simulink model "CurrentSystem2019a"  (R2019a)
settings: Solver=ode23tb  StartTime=0  StopTime=24*365*60*60  RelTol=0.1  EnableMultiTasking=on
PreLoadFcn:
  | power_13NodeTestFeeder_init;
undefined symbols (not defined in the file): ABSOLARCap, ABWindCap, BCSOLARCap, BCWindCap, C_601, C_602, C_603, C_604, C_605, C_606, C_607, ft2km, L_601, L_602, L_603, L_604, L_605, L_606, L_607, MBSOLARCap, MBWindCap, NBSOLARCap, NBWindCap, NLSOLARCap, NLWindCap, NSSOLARCap, NSWindCap, NTSOLARCap, NTWindCap, NUSOLARCap, NUWindCap, ONSOLARCap, ONWindCap, PEISOLARCap, PEIWindCap, QCSOLARCap, QCWindCap, R_601, R_602, R_603, R_604, R_605, R_606, R_607, SKSOLARCap, SKWindCap, T_Disconnect, T_Reconnect, Yearsec, YTSOLARCap, YTWindCap
libraries: powerlib_meascontrol x70, powerlib x67, sps_avr x1, spsDieselMotorModel x1
(part 1 of 3)
settings Model: SimulationMode=accelerator  Creator=MathWorks  LastModifiedBy=100618997
settings SolverCC: ZeroCrossControl=DisableAll  ZeroCrossAlgorithm=Adaptive
settings DataIOCC: ExternalInput=getinputstruct(op_IEEE_13_node_5)  InitialState=getstatestruct(op_IEEE_13_node_5)  LimitDataPoints=on  SaveFormat=Array  SaveOutput=off  SignalLogging=off  DSMLogging=off  SaveTime=off  ReturnWorkspaceOutputs=off
settings OptimizationCC: ExpressionDepthLimit=2147483647  EfficientMapNaN2IntZero=off  LifeSpan=inf
settings DebuggingCC: ReadBeforeWriteMsg=DisableAll  WriteAfterWriteMsg=DisableAll  WriteAfterReadMsg=DisableAll  AlgebraicLoopMsg=none  UnderspecifiedInitializationDetection=Classic  MergeDetectMultiDrivingBlocksExec=none  MultiTaskDSMMsg=none  FcnCallInpInsideContextMsg=warning  UnconnectedInputMsg=none  UnconnectedOutputMsg=none  UnconnectedLineMsg=none  AllowSymbolicDim=off  StateNameClashWarn=warning  SFUnexpectedBacktrackingDiag=warning  SFNoUnconditionalDefaultTransitionDiag=warning  SFExecutionAtInitializationDiag=none  ArithmeticOperatorsInVariantConditions=warning
settings HardwareCC: ProdBitPerPointer=32  ProdBitPerSizeT=32  ProdBitPerPtrDiffT=32  ProdLargestAtomicFloat=None  ProdIntDivRoundTo=Undefined  ProdEndianess=Unspecified  ProdWordSize=32  ProdHWDeviceType=32-bit Generic  TargetBitPerPointer=64  TargetBitPerSizeT=64  TargetBitPerPtrDiffT=64  TargetLongLongMode=on  TargetIntDivRoundTo=Zero  TargetEndianess=LittleEndian  TargetWordSize=64  TargetHWDeviceType=MATLAB Host  ProdEqTarget=off
settings ModelReferenceCC: PropagateSignalLabelsOutOfModel=off
settings SFSimCC: SFSimEcho=off  SimUseLocalCustomCode=off
settings CodeAppCC: MaxIdLength=128
settings GRTTargetCC: TargetLangStandard=C89/C90 (ANSI)  GRTInterface=on
settings ConfigComp: CovMetricSettings=dw  CovHtmlReporting=on  CovSaveCumulativeToWorkspaceVar=on  CovSaveSingleToWorkspaceVar=on  CovExternalEMLEnable=off  CovSFcnEnable=off
settings SimscapeCC: SimscapeNormalizeSystem=off

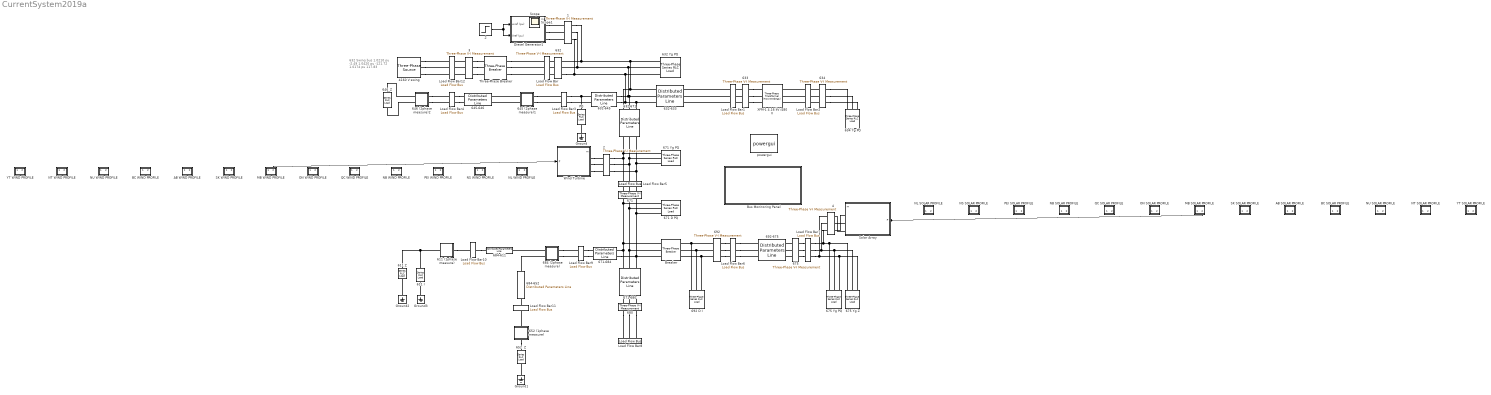
== system CurrentSystem2019a ==
  note: 632 Swing bus
      | 1.0210 pu -2.49
      | 1.0420 pu -121.72
      | 1.0174 pu 117.83
  " 634 Yg PQ " : powerlib/Elements/Three-Phase Series RLC Load  LConnTagsString=A|B|C  Configuration=Y (grounded)  NominalVoltage=120e3  Vabc=[ 0.991722 1.02022 0.993738]*277.128  Vabcp=[1e3 1e3 1e3]  NominalFrequency=60  UnbalancedPower=on  ActivePower=1e+006  InductivePower=0  CapacitivePower=0  Pabc=[160 120 120]*1e3  QLabc=[110 90 90]*1e3  QCabc=[0 0 0]  Pabcp=[10e3 9e3 11e3]  QLabcp=[100 90 110]  QCabcp=[100 90 110]  Measurements=None  LoadType=constant PQ
      settings: SourceProductName=Simscape Electrical
      settings: AttributesFormatString=|
      | P= %<Pabc> W
      | Ql=%<QLabc> var
      | Qc=%<QCabc> var
  .2 : Step  Time=T_Reconnect  Before=1  After=0  SampleTime=0
  1 : powerlib/Measurements/Three-Phase V-I Measurement  VoltageMeasurement=phase-to-ground  SetLabelV=on  LabelV=Vdiesel  Vpu=off  VpuLL=off  CurrentMeasurement=yes  SetLabelI=on  LabelI=Idiesel  Ipu=off  Pbase=100e6  Vbase=4160  OutputType=Complex  PhasorSimulation=on  PSBequivalent=0
      settings: SourceProductName=Simscape Electrical
  2 : powerlib/Measurements/Three-Phase V-I Measurement  VoltageMeasurement=phase-to-ground  SetLabelV=on  LabelV=Vwind  Vpu=off  VpuLL=off  CurrentMeasurement=yes  SetLabelI=on  LabelI=Iwind  Ipu=off  Pbase=100e6  Vbase=4160  OutputType=Complex  PhasorSimulation=on  PSBequivalent=0
      settings: SourceProductName=Simscape Electrical
  3 : powerlib/Measurements/Three-Phase V-I Measurement  VoltageMeasurement=phase-to-ground  SetLabelV=on  LabelV=Vmaingrid  Vpu=off  VpuLL=off  CurrentMeasurement=yes  SetLabelI=on  LabelI=Imaingrid  Ipu=off  Pbase=100e6  Vbase=4160  OutputType=Complex  PhasorSimulation=on  PSBequivalent=0
      settings: SourceProductName=Simscape Electrical
  4 : powerlib/Measurements/Three-Phase V-I Measurement  VoltageMeasurement=phase-to-ground  SetLabelV=on  LabelV=Vsolar  Vpu=off  VpuLL=off  CurrentMeasurement=yes  SetLabelI=on  LabelI=Isolar  Ipu=off  Pbase=100e6  Vbase=4160  OutputType=Complex  PhasorSimulation=on  PSBequivalent=0
      settings: SourceProductName=Simscape Electrical
  4160 V swing : powerlib/Electrical Sources/Three-Phase Source  InternalConnection=Yg  VoltagePhases=on  Voltage=120e3  PhaseAngle=0  Voltage_phases=[ 1.021 1.042 1.0174]*2401.78  PhaseAngles_phases=[ -2.49 -121.72 117.83]  Frequency=60  NonIdealSource=off  SpecifyImpedance=on  Resistance=0.8929  Inductance=16.58e-3  ShortCircuitLevel=100e6  BaseVoltage=120e3  XRratio=10  BusType=swing  Pref=0  Qref=0  Prefabc=[1 1 1]*1e6  Qrefabc=[0 0 0]  Qmin="[-inf  -inf -inf]"  Qmax="[inf  inf inf]"
      settings: SourceProductName=Simscape Electrical
  611 (1phase measure) : Subsystem
  611 I : powerlib/Elements/Series RLC Load  LConnTagsString=a  RConnTagsString=__new0  NominalVoltage=0.985825*2401.78  NominalFrequency=60  ActivePower=170e3  InductivePower=80e3  CapacitivePower=0  Setx0=off  InitialVoltage=0  SetiL0=off  InitialCurrent=0  Measurements=Branch voltage and current  LoadType=constant I
      settings: SourceProductName=Simscape Electrical
      settings: AttributesFormatString=|
      | P=%<ActivePower> W
      | Ql=%<InductivePower> var
      | Qc=%<CapacitivePower> var
  611 Z : powerlib/Elements/Series RLC Load  LConnTagsString=a  RConnTagsString=__new0  NominalVoltage=4160/sqrt(3)  NominalFrequency=60  ActivePower=0  InductivePower=0  CapacitivePower=100e3  Setx0=off  InitialVoltage=0  SetiL0=off  InitialCurrent=0  Measurements=None  LoadType=constant Z
      settings: SourceProductName=Simscape Electrical
      settings: AttributesFormatString=|
      | P=%<ActivePower> W
      | Ql=%<InductivePower> var
      | Qc=%<CapacitivePower> var
  632 : powerlib/Measurements/Three-Phase V-I Measurement  VoltageMeasurement=phase-to-ground  SetLabelV=on  LabelV=Vabc_632  Vpu=off  VpuLL=off  CurrentMeasurement=yes  SetLabelI=on  LabelI=Iabc_632  Ipu=off  Pbase=100e6  Vbase=4160  OutputType=Complex  PhasorSimulation=on  PSBequivalent=0
      settings: SourceProductName=Simscape Electrical
  632 Yg PQ : powerlib/Elements/Three-Phase Series RLC Load  LConnTagsString=A|B|C  Configuration=Y (grounded)  NominalVoltage=120e3  Vabc=[ 1.01897 1.04044 1.01532]*2401.78  Vabcp=[1e3 1e3 1e3]  NominalFrequency=60  UnbalancedPower=on  ActivePower=1e+006  InductivePower=0  CapacitivePower=0  Pabc="[17 66  117]*1e3/2"  QLabc="[10 38  68]*1e3/2"  QCabc=[0 0 0]  Pabcp=[10e3 9e3 11e3]  QLabcp=[100 90 110]  QCabcp=[100 90 110]  Measurements=None  LoadType=constant PQ
      settings: SourceProductName=Simscape Electrical
      settings: AttributesFormatString=|
      | P= %<Pabc> W
      | Ql=%<QLabc> var
      | Qc=%<QCabc> var
  632-633 : powerlib/Elements/Distributed Parameters Line  Phases=3  Frequency=60  Resistance=R_602  Inductance=L_602  Capacitance=C_602  Length=500*ft2km  x1=[501.298249556744 4241.38280163391 4282.12708189344;376.991118430775 376.991118430775 376.991118430775;-2.2614148733286 -0.34157510745785 -1.9168137180942]  x2=[504.588684561712 4230.72062513662 4271.71287268223;376.991118430775 376.991118430775 376.991118430775;-2.26353543885085 -0.342275768758346 -1.91742725559162]  x3=[16.7674456646186 117.682569324759 103.368907043517;376.991118430775 376.991118430775 376.991118430775;2.65069587435361 2.14578500124131 0.446625957105985]  x4=[16.5551069121651 140.665410457147 120.655553593327;376.991118430775 376.991118430775 376.991118430775;-0.568878729363739 -0.875843142008242 -2.56215385674791]  x5=6.41053351781503e-07  V1=ones(3,3)  V2=ones(3,3)  I1=ones(3,3)  I2=ones(3,3)  nHarmo=1  Measurements=None
      settings: SourceProductName=Simscape Electrical
  632-645 : powerlib/Elements/Distributed Parameters Line  Phases=2  Frequency=60  Resistance=R_603(2:3,2:3)  Inductance=L_603(2:3,2:3)  Capacitance=C_603(2:3,2:3)  Length=500*ft2km  x1=[4264.40256081592 2449.37120000517;376.991118430775 376.991118430775;-1.61351597014441 3.12257330541687]  x2=[4292.15394533527 2455.18167402023;376.991118430775 376.991118430775;-1.614116105248 3.12994263723761]  x3=[213.394300129666 87.8697003438014;376.991118430775 376.991118430775;-2.34443706998439 -2.78105546765574]  x4=[197.96033050634 81.3060039726639;376.991118430775 376.991118430775;0.724911523434161 0.392615068886907]  x5=6.57914367465262e-07  V1=ones(3,3)  V2=ones(3,3)  I1=ones(3,3)  I2=ones(3,3)  nHarmo=1  Measurements=None
      settings: SourceProductName=Simscape Electrical
  632-671 : powerlib/Elements/Distributed Parameters Line  Phases=3  Frequency=60  Resistance=R_601  Inductance=L_601  Capacitance=C_601  Length=2000*ft2km  x1=[411.258072802617 4262.34154212984 4279.413254268;376.991118430775 376.991118430775 376.991118430775;2.58888404049218 0.275850406288993 1.83441514058537]  x2=[346.273446515285 4158.03643956185 4231.93277610758;376.991118430775 376.991118430775 376.991118430775;2.89883497125866 0.262414212273929 1.80030975234441]  x3=[177.438259148728 550.32580669605 566.66947309912;376.991118430775 376.991118430775 376.991118430775;-2.70857378445777 2.65722725515321 -1.37114447017259]  x4=[176.777093380408 575.063462206073 592.863838960838;376.991118430775 376.991118430775 376.991118430775;0.437240559698923 -0.444758677085734 1.77250930915245]  x5=2.51909782126786e-06  V1=ones(3,3)  V2=ones(3,3)  I1=ones(3,3)  I2=ones(3,3)  nHarmo=1  Measurements=None
      settings: SourceProductName=Simscape Electrical
  633 : powerlib/Measurements/Three-Phase V-I Measurement  VoltageMeasurement=phase-to-ground  SetLabelV=on  LabelV=Vabc_633  Vpu=off  VpuLL=off  CurrentMeasurement=yes  SetLabelI=on  LabelI=Iabc_633  Ipu=off  Pbase=100e6  Vbase=4160  OutputType=Complex  PhasorSimulation=on  PSBequivalent=0
      settings: SourceProductName=Simscape Electrical
  634 : powerlib/Measurements/Three-Phase V-I Measurement  VoltageMeasurement=phase-to-ground  SetLabelV=on  LabelV=Vabc_634  Vpu=off  VpuLL=off  CurrentMeasurement=yes  SetLabelI=on  LabelI=Iabc_634  Ipu=off  Pbase=100e6  Vbase=4160  OutputType=Complex  PhasorSimulation=on  PSBequivalent=0
      settings: SourceProductName=Simscape Electrical
  645 (2phase measure)1 : Subsystem
  645-646 : powerlib/Elements/Distributed Parameters Line  Phases=2  Frequency=60  Resistance=R_603(2:3,2:3)  Inductance=L_603(2:3,2:3)  Capacitance=C_603(2:3,2:3)  Length=300*ft2km  x1=[4253.51615943753 2449.23478756666;376.991118430775 376.991118430775;1.53247826718143 3.11934493784883]  x2=[4264.00783705366 2449.21160966797;376.991118430775 376.991118430775;1.53284927772704 3.11937264911809]  x3=[139.76322829713 3.84735914896354;376.991118430775 376.991118430775;1.04719191601338 -3.04482503601123]  x4=[121.315610473818 3.30490803236315;376.991118430775 376.991118430775;-2.17648289094728 2.98054667861466]  x5=3.94748620479157e-07  V1=ones(3,3)  V2=ones(3,3)  I1=ones(3,3)  I2=ones(3,3)  nHarmo=1  Measurements=None
      settings: SourceProductName=Simscape Electrical
  646 (2phase measure)2 : Subsystem
  646_Z : powerlib/Elements/Series RLC Load  LConnTagsString=a  RConnTagsString=__new0  NominalVoltage=4160  NominalFrequency=60  ActivePower=230e3  InductivePower=132e3  CapacitivePower=0  Setx0=off  InitialVoltage=0  SetiL0=off  InitialCurrent=0  Measurements=None  LoadType=constant Z
      settings: SourceProductName=Simscape Electrical
      settings: AttributesFormatString=|
      | P=%<ActivePower> W
      | Ql=%<InductivePower> var
      | Qc=%<CapacitivePower> var
  "652  Z " : powerlib/Elements/Series RLC Load  LConnTagsString=a  RConnTagsString=__new0  NominalVoltage=4160/sqrt(3)  NominalFrequency=60  ActivePower=128e3  InductivePower=86e3  CapacitivePower=0  Setx0=off  InitialVoltage=0  SetiL0=off  InitialCurrent=0  Measurements=None  LoadType=constant Z
      settings: SourceProductName=Simscape Electrical
      settings: AttributesFormatString=|
      | P=%<ActivePower> W
      | Ql=%<InductivePower> var
      | Qc=%<CapacitivePower> var
  652 (1phase measure) : Subsystem
  671 : powerlib/Measurements/Three-Phase V-I Measurement  VoltageMeasurement=phase-to-ground  SetLabelV=on  LabelV=Vabc_671  Vpu=off  VpuLL=off  CurrentMeasurement=yes  SetLabelI=on  LabelI=Iabc_671  Ipu=off  Pbase=100e6  Vbase=4160  OutputType=Complex  PhasorSimulation=on  PSBequivalent=0
      settings: SourceProductName=Simscape Electrical
  671 D PQ : powerlib/Elements/Three-Phase Series RLC Load  LConnTagsString=A|B|C  Configuration=Delta  NominalVoltage=120e3  Vabc="[1  1  1]*120e3/sqrt(3)"  Vabcp=[ 1.73966 1.76988 1.71151]*2401.78  NominalFrequency=60  UnbalancedPower=on  ActivePower=1e+006  InductivePower=0  CapacitivePower=0  Pabc="[17 66  117]*1e3/2"  QLabc="[10 38  68]*1e3/2"  QCabc=[0 0 0]  Pabcp=[385 385 385 ]*1e3  QLabcp=[220 220 220]*1e3  QCabcp="[0  0  0]"  Measurements=Branch voltages and currents  LoadType=constant PQ
      settings: SourceProductName=Simscape Electrical
      settings: AttributesFormatString=|
      | P= %<Pabcp> W
      | Ql=%<QLabcp> var
      | Qc=%<QCabcp> var
  671 Yg PQ : powerlib/Elements/Three-Phase Series RLC Load  LConnTagsString=A|B|C  Configuration=Y (grounded)  NominalVoltage=120e3  Vabc=[ 0.987901 1.05099 0.975851]*2401.78  Vabcp=[1e3 1e3 1e3]  NominalFrequency=60  UnbalancedPower=on  ActivePower=1e+006  InductivePower=0  CapacitivePower=0  Pabc="[17 66  117]*1e3/2"  QLabc="[10 38  68]*1e3/2"  QCabc=[0 0 0]  Pabcp=[10e3 9e3 11e3]  QLabcp=[100 90 110]  QCabcp=[100 90 110]  Measurements=None  LoadType=constant PQ
      settings: SourceProductName=Simscape Electrical
      settings: AttributesFormatString=|
      | P= %<Pabc> W
      | Ql=%<QLabc> var
      | Qc=%<QCabc> var
  671-680 : powerlib/Elements/Distributed Parameters Line  Phases=3  Frequency=60  Resistance=R_601  Inductance=L_601  Capacitance=C_601  Length=1000*ft2km  x1=[346.273446515285 4158.03643956185 4231.93277610758;376.991118430775 376.991118430775 376.991118430775;2.8993098100112 0.262807128835779 1.80070073244037]  x2=[346.273485552757 4158.03676052785 4231.93309956574;376.991118430775 376.991118430775 376.991118430775;2.89930977124762 0.262807101445064 1.80070071123254]  x3=[0.46178374393002 16.4417222910227 13.0406156867181;376.991118430775 376.991118430775 376.991118430775;2.89883495201253 0.262414198558244 1.80030974173376]  x4=[0.461783743355683 16.4417222911636 13.0406156869002;376.991118430775 376.991118430775 376.991118430775;2.89930977111503 0.262807101464808 1.80070071123926]  x5=1.25954891063393e-06  V1=ones(3,3)  V2=ones(3,3)  I1=ones(3,3)  I2=ones(3,3)  nHarmo=1  Measurements=None
      settings: SourceProductName=Simscape Electrical
  671-684 : powerlib/Elements/Distributed Parameters Line  Phases=2  Frequency=60  Resistance=R_604([1 3],[1 3])  Inductance=L_604([1 3],[1 3])  Capacitance=C_604([1 3],[1 3])  Length=300*ft2km  x1=[2317.38621246171 4117.96109624564;376.991118430775 376.991118430775;0.961696703414869 2.54346818296187]  x2=[2319.24198937793 4127.84304358144;376.991118430775 376.991118430775;0.96282674091554 2.54452459092107]  x3=[27.1884655613009 142.758498027598;376.991118430775 376.991118430775;1.03773453761655 2.30448005568221]  x4=[20.4997438318642 122.806338198603;376.991118430775 376.991118430775;-2.07913574984399 -0.876981828337958]  x5=3.94748620479157e-07  V1=ones(3,3)  V2=ones(3,3)  I1=ones(3,3)  I2=ones(3,3)  nHarmo=1  Measurements=None
      settings: SourceProductName=Simscape Electrical
  "675 " : powerlib/Measurements/Three-Phase V-I Measurement  VoltageMeasurement=phase-to-ground  SetLabelV=on  LabelV=Vabc_675  Vpu=off  VpuLL=off  CurrentMeasurement=yes  SetLabelI=on  LabelI=Iabc_675  Ipu=off  Pbase=100e6  Vbase=4160  OutputType=Complex  PhasorSimulation=on  PSBequivalent=0
      settings: SourceProductName=Simscape Electrical
  675 Yg PQ : powerlib/Elements/Three-Phase Series RLC Load  LConnTagsString=A|B|C  Configuration=Y (grounded)  NominalVoltage=120e3  Vabc=[ 0.98146 1.05342 0.973762]*2401.78  Vabcp=[1e3 1e3 1e3]  NominalFrequency=60  UnbalancedPower=on  ActivePower=1e+006  InductivePower=0  CapacitivePower=0  Pabc="[485  68  290]*1e3"  QLabc="[190  60  212]*1e3"  QCabc=[0 0 0]  Pabcp=[10e3 9e3 11e3]  QLabcp=[100 90 110]  QCabcp=[100 90 110]  Measurements=Branch voltages and currents  LoadType=constant PQ
      settings: SourceProductName=Simscape Electrical
      settings: AttributesFormatString=|
      | P= %<Pabc> W
      | Ql=%<QLabc> var
      | Qc=%<QCabc> var
  675 Yg Z : powerlib/Elements/Three-Phase Series RLC Load  LConnTagsString=A|B|C  Configuration=Y (grounded)  NominalVoltage=120e3  Vabc="[1  1  1]*4160/sqrt(3)"  Vabcp=[1e3 1e3 1e3]  NominalFrequency=60  UnbalancedPower=on  ActivePower=1e+006  InductivePower=0  CapacitivePower=0  Pabc=[0 0 0]  QLabc=[0 0 0]  QCabc=[200 200 200]*1e3  Pabcp=[10e3 9e3 11e3]  QLabcp=[100 90 110]  QCabcp=[100 90 110]  Measurements=None  LoadType=constant Z
      settings: SourceProductName=Simscape Electrical
      settings: AttributesFormatString=|
      | P= %<Pabc> W
      | Ql=%<QLabc> var
      | Qc=%<QCabc> var
  680 : powerlib/Measurements/Three-Phase V-I Measurement  VoltageMeasurement=phase-to-ground  SetLabelV=on  LabelV=Vabc_680  Vpu=off  VpuLL=off  CurrentMeasurement=yes  SetLabelI=on  LabelI=Iabc_680  Ipu=off  Pbase=100e6  Vbase=4160  OutputType=Complex  PhasorSimulation=on  PSBequivalent=0
      settings: SourceProductName=Simscape Electrical
  684 (2phase measure) : Subsystem
  684-611 : powerlib/Elements/Distributed Parameters Line  Phases=1  Frequency=60  Resistance=R_605(3,3)  Inductance=L_605(3,3)  Capacitance=C_605(3,3)  Length=300*ft2km  x1=[3314.5063708128;376.991118430775;2.02689942323022]  x2=[3321.32988758383;376.991118430775;2.02944736803624]  x3=[107.053862067257;376.991118430775;2.12194507149989]  x4=[94.9628871920728;376.991118430775;-1.00765726793177]  x5=3.71926621942778e-07  V1=ones(3,3)  V2=ones(3,3)  I1=ones(3,3)  I2=ones(3,3)  nHarmo=1  Measurements=None
      settings: SourceProductName=Simscape Electrical
  684-652 : powerlib/Elements/Distributed Parameters Line  Phases=1  Frequency=60  Resistance=R_607(1,1)  Inductance=L_607(1,1)  Capacitance=C_607(1,1)  Length=800*ft2km  x1=[3364.00980712148;376.991118430775;-0.0876071344539785]  x2=[3345.0390998936;376.991118430775;-0.0863060663875372]  x3=[57.9909734563849;376.991118430775;2.02581298772652]  x4=[128.189096775588;376.991118430775;-0.48531897158013]  x5=2.71396421650751e-06  V1=ones(3,3)  V2=ones(3,3)  I1=ones(3,3)  I2=ones(3,3)  nHarmo=1  Measurements=None
      settings: SourceProductName=Simscape Electrical
  692 : powerlib/Measurements/Three-Phase V-I Measurement  VoltageMeasurement=phase-to-ground  SetLabelV=on  LabelV=Vabc_692  Vpu=off  VpuLL=off  CurrentMeasurement=yes  SetLabelI=on  LabelI=Iabc_692  Ipu=off  Pbase=100e6  Vbase=4160  OutputType=Complex  PhasorSimulation=on  PSBequivalent=0
      settings: SourceProductName=Simscape Electrical
  692 D I : powerlib/Elements/Three-Phase Series RLC Load  LConnTagsString=A|B|C  Configuration=Delta  NominalVoltage=120e3  Vabc="[1  1  1]*120e3/sqrt(3)"  Vabcp=[ 1.73585 1.75086 1.72174]*2401.78  NominalFrequency=60  UnbalancedPower=on  ActivePower=1e+006  InductivePower=0  CapacitivePower=0  Pabc="[17 66  117]*1e3/2"  QLabc="[10 38  68]*1e3/2"  QCabc=[0 0 0]  Pabcp=[1e-6 1e-6 170 ]*1e3  QLabcp=[0 0 151]*1e3  QCabcp="[0  0  0]"  Measurements=Branch voltages and currents  LoadType=constant I
      settings: SourceProductName=Simscape Electrical
      settings: AttributesFormatString=|
      | P= %<Pabcp> W
      | Ql=%<QLabcp> var
      | Qc=%<QCabcp> var
  692-675 : powerlib/Elements/Distributed Parameters Line  Phases=3  Frequency=60  Resistance=R_606  Inductance=L_606  Capacitance=C_606  Length=500*ft2km  x1=[241.289496642843 4129.29083181281 4257.51535779195;376.991118430775 376.991118430775 376.991118430775;-1.71976827629363 2.54633306210785 -2.14602940424835]  x2=[256.665851258922 4119.5124518439 4255.36005403233;376.991118430775 376.991118430775 376.991118430775;-1.79076499561998 2.54378648977405 -2.14685741555792]  x3=[166.881820949653 164.603040297361 23.9250117588126;376.991118430775 376.991118430775 376.991118430775;-2.92243066280774 -0.42985333149663 2.52484844339319]  x4=[164.240261344418 287.086932785949 139.040045332788;376.991118430775 376.991118430775 376.991118430775;0.179837319068752 2.64019694933151 -1.97394240629806]  x5=1.72234634931087e-06  V1=ones(3,3)  V2=ones(3,3)  I1=ones(3,3)  I2=ones(3,3)  nHarmo=1  Measurements=None
      settings: SourceProductName=Simscape Electrical
  AB SOLAR PROFILE : Subsystem
  AB WIND PROFILE : Subsystem
  BC SOLAR PROFILE : Subsystem
  BC WIND PROFILE : Subsystem
  Breaker : powerlib/Elements/Three-Phase Breaker  InitialState=closed  SwitchA=off  SwitchB=off  SwitchC=off  SwitchTimes=[0.5 ]  External=off  BreakerResistance=0.0001  SnubberResistance=inf  SnubberCapacitance=0  Measurements=None
      settings: SourceProductName=Simscape Electrical
  Bus Monitoring Panel : Subsystem
  Diesel Generator1 : Subsystem  mask(Diesel Generator (Simple)){Pn=3e6, Vn=4160, Fn=60, genType=PQ, PQ0=[0 0]}
      mask prompts: Pn "Generator Rated Power [W]"; Vn "Rated Voltage [V]"; Fn "Rated Frequency [Hz]"; genType "Load Flow Type"; PQ0 "Initial Power, [P0 Q0] [pu]"
      mask help:
      | The Diesel Generator block contains a synchronous generator, diesel governor and excitation system to represent the dynamics of a Genset. To inspect the model, look under the block mask (Ctrl + u).
      |
      | The inputs to the basic Diesel generator block are the desired speed reference (in pu) and the desired voltage reference (in pu). The output measurements are contained in a Simulink bus, which can be selected by using the Bus Selector block.
      |
      | Note: The initial generator power must be specified for use for Load Flow analysis.
      mask init:
      | % Extract Initial Active/Reactive Power
      | P0 = PQ0(1);
      | Q0 = PQ0(2);
      | 
      | % Select Load Flow Type
      | genBlock = [gcb '/Synchronous Machine'];
      | currentVals = get_param(genBlock,'MaskValues');
      | currentVals{31} = genType;
      | set_param(genBlock,'MaskValues',currentVals);
      | 
      | % Disable Option if Swing Generator Selected
      | currentEnables = get_param(gcb,'MaskEnables');
      | if strcmp(genType,'swing')
      |     currentEnables{5} = 'off';
      | else
      |     currentEnables{5} = 'on';
      | end
      | set_param(gcb,'MaskEnables',currentEnables);
      settings: AttributesFormatString=Rated Power: %<Pn> W
      mask TypeOptions genType: swing | PQ | PV
      mask Display: %image(imread('diesel.jpg'))
  Ground{,1..3} (4 alike) : powerlib/Elements/Ground  LConnTagsString=a
      settings: SourceProductName=Simscape Electrical
  Load Flow Bar : powerlib/Measurements/Load Flow Bus  LConnTagsString=a|b|c  RConnTagsString=a|b|c  Phases=ABC  Connectors=on both sides  ID=632  Vbase=4160/sqrt(3)  Vref="[ 1.0210  1.0420  1.0174]"  Vangle="[ -2.49  -121.72  117.83]"  VLF=1.019  VLFb=1.04  VLFc=1.015  angleLF=-2.435  angleLFb=-121.7  angleLFc=117.9
      settings: AttributesFormatString=%<ID>  SourceProductName=Simscape Electrical
  Load Flow Bar1 : powerlib/Measurements/Load Flow Bus  LConnTagsString=a|b|c  RConnTagsString=a|b|c  Phases=ABC  Connectors=on both sides  ID=633  Vbase=4160/sqrt(3)  Vref=[1.0 1.0 1.0]  Vangle=[0 -120 120]  VLF=1.016  VLFb=1.039  VLFc=1.013  angleLF=-2.504  angleLFb=-121.7  angleLFc=117.9
      settings: AttributesFormatString=%<ID>  SourceProductName=Simscape Electrical
  Load Flow Bar10 : powerlib/Measurements/Load Flow Bus  LConnTagsString=a  RConnTagsString=a  Phases=C  Connectors=on both sides  ID=611  Vbase=4160/sqrt(3)  Vref=1.0  Vangle=0  VLF=NaN  VLFb=NaN  VLFc=0.9719  angleLF=NaN  angleLFb=NaN  angleLFc=115.8
      settings: AttributesFormatString=%<ID>  SourceProductName=Simscape Electrical
  Load Flow Bar11 : powerlib/Measurements/Load Flow Bus  LConnTagsString=a  RConnTagsString=a  Phases=A  Connectors=on both sides  ID=652  Vbase=4160/sqrt(3)  Vref=1.0  Vangle=0  VLF=0.9804  VLFb=NaN  VLFc=NaN  angleLF=-5.174  angleLFb=NaN  angleLFc=NaN
      settings: AttributesFormatString=%<ID>  SourceProductName=Simscape Electrical
  Load Flow Bar12 : powerlib/Measurements/Load Flow Bus  LConnTagsString=a|b|c  RConnTagsString=a|b|c  Phases=ABC  Connectors=on both sides  ID=MAINGRID  Vbase=4160/sqrt(3)  Vref="[ 1.0210  1.0420  1.0174]"  Vangle="[ -2.49  -121.72  117.83]"  VLF=1.021  VLFb=1.042  VLFc=1.017  angleLF=-2.49  angleLFb=-121.7  angleLFc=117.8
      settings: AttributesFormatString=%<ID>  SourceProductName=Simscape Electrical
  Load Flow Bar2 : powerlib/Measurements/Load Flow Bus  LConnTagsString=a|b|c  RConnTagsString=a|b|c  Phases=ABC  Connectors=on both sides  ID=634  Vbase=480/sqrt(3)  Vref=[1.0 1.0 1.0]  Vangle=[0 -120 120]  VLF=0.9917  VLFb=1.02  VLFc=0.9937  angleLF=-3.184  angleLFb=-122.2  angleLFc=117.4
      settings: AttributesFormatString=%<ID>  SourceProductName=Simscape Electrical
  Load Flow Bar3 : powerlib/Measurements/Load Flow Bus  LConnTagsString=a|b  RConnTagsString=a|b  Phases=BC  Connectors=on both sides  ID=645  Vbase=4160/sqrt(3)  Vref=[1.0 1.0 ]  Vangle=[0 0]  VLF=NaN  VLFb=1.031  VLFc=1.013  angleLF=NaN  angleLFb=-121.9  angleLFc=117.9
      settings: AttributesFormatString=%<ID>  SourceProductName=Simscape Electrical
  Load Flow Bar4 : powerlib/Measurements/Load Flow Bus  LConnTagsString=a|b  RConnTagsString=a|b  Phases=BC  Connectors=on both sides  ID=646  Vbase=4160/sqrt(3)  Vref=[1.0 1.0 ]  Vangle=[0 0]  VLF=NaN  VLFb=1.011  VLFc=1.03  angleLF=NaN  angleLFb=118  angleLFc=-121.9
      settings: AttributesFormatString=%<ID>  SourceProductName=Simscape Electrical
  Load Flow Bar5 : powerlib/Measurements/Load Flow Bus  LConnTagsString=a|b|c  RConnTagsString=a|b|c  Phases=ABC  Connectors=on both sides  ID=671  Vbase=4160/sqrt(3)  Vref=[1.0 1.0 1.0]  Vangle=[0 -120 120]  VLF=0.9879  VLFb=1.051  VLFc=0.9759  angleLF=-5.226  angleLFb=-122.3  angleLFc=116.1
      settings: AttributesFormatString=%<ID>  SourceProductName=Simscape Electrical
  Load Flow Bar6 : powerlib/Measurements/Load Flow Bus  LConnTagsString=a|b|c  RConnTagsString=a|b|c  Phases=ABC  Connectors=on both sides  ID=692  Vbase=4160/sqrt(3)  Vref=[1.0 1.0 1.0]  Vangle=[0 -120 120]  VLF=0.9879  VLFb=1.051  VLFc=0.9758  angleLF=-5.226  angleLFb=-122.3  angleLFc=116.1
      settings: AttributesFormatString=%<ID>  SourceProductName=Simscape Electrical
  Load Flow Bar7 : powerlib/Measurements/Load Flow Bus  LConnTagsString=a|b|c  RConnTagsString=a|b|c  Phases=ABC  Connectors=on both sides  ID=675  Vbase=4160/sqrt(3)  Vref=[1.0 1.0 1.0]  Vangle=[0 -120 120]  VLF=0.9815  VLFb=1.053  VLFc=0.9738  angleLF=-5.471  angleLFb=-122.5  angleLFc=116.1
      settings: AttributesFormatString=%<ID>  SourceProductName=Simscape Electrical
  Load Flow Bar8 : powerlib/Measurements/Load Flow Bus  LConnTagsString=a|b|c  Phases=ABC  Connectors=on one side  ID=680  Vbase=4160/sqrt(3)  Vref=[1.0 1.0 1.0]  Vangle=[0 -120 120]  VLF=0.9879  VLFb=1.051  VLFc=0.9759  angleLF=-5.226  angleLFb=-122.3  angleLFc=116.1
      settings: AttributesFormatString=%<ID>  SourceProductName=Simscape Electrical
  Load Flow Bar9 : powerlib/Measurements/Load Flow Bus  LConnTagsString=a|b  RConnTagsString=a|b  Phases=AC  Connectors=on both sides  ID=684  Vbase=4160/sqrt(3)  Vref=[1.0 1.0 ]  Vangle=[0 -120 ]  VLF=0.986  VLFb=NaN  VLFc=0.9739  angleLF=-5.249  angleLFb=NaN  angleLFc=116
      settings: AttributesFormatString=%<ID>  SourceProductName=Simscape Electrical
  MB SOLAR PROFILE : Subsystem
  MB WIND PROFILE : Subsystem
  NB SOLAR PROFILE : Subsystem
  NB WIND PROFILE : Subsystem
  NL SOLAR PROFILE : Subsystem
  NL WIND PROFILE : Subsystem
  NS SOLAR PROFILE : Subsystem
  NS WIND PROFILE : Subsystem
  NT SOLAR PROFILE : Subsystem
  NT WIND PROFILE : Subsystem
  NU SOLAR PROFILE : Subsystem
  NU WIND PROFILE : Subsystem
  ON SOLAR PROFILE : Subsystem
  ON WIND PROFILE : Subsystem
  PEI SOLAR PROFILE : Subsystem
  PEI WIND PROFILE : Subsystem
  PQ : powerlib/Elements/Series RLC Load  LConnTagsString=a  RConnTagsString=__new0  NominalVoltage=1.03133*2401.78  NominalFrequency=60  ActivePower=170e3  InductivePower=125e3  CapacitivePower=0  Setx0=off  InitialVoltage=0  SetiL0=off  InitialCurrent=0  Measurements=None  LoadType=constant PQ
      settings: SourceProductName=Simscape Electrical
      settings: AttributesFormatString=|
      | P=%<ActivePower> W
      | Ql=%<InductivePower> var
      | Qc=%<CapacitivePower> var
  QC SOLAR PROFILE : Subsystem
  QC WIND PROFILE : Subsystem
  SK SOLAR PROFILE : Subsystem
  SK WIND PROFILE : Subsystem
  Solar Array : Subsystem  mask(Grid-Connected PV Array (PQ Model)){Vn=4160, Fn=60, P0=.05*4000e3}
      mask prompts: Vn "Nominal L-L Voltage [Vrms]"; Fn "Nominal Frequency [Hz]"; P0 "Initial Power [W]"
      mask help:
      | This block models a grid-connected solar array using the Three-Phase Dynamic Load block. This is a system-level model that does not contain any power electronics, but is useful for load flow, phasor, and hybrid phasor-EMT simulations. The input to this block is the power output of the grid connected PV array, not irradiance.
      |
      | For more detailed PV models, consider the PV Array block in the Renewables library. Consider using this PQ Model to perform load flow studies and switch to a more detailed model when full EMT studies are required.
      |
      | Note: The array power must be specified for use for Load Flow analysis.
      mask init:
      | % P0 = Irr0*TotalArea*Efficiency/100;
      | P0 = -P0;
      mask Display:
      | image(imread('PV_Farm.jpg'))
      | color('white')
      | port_label('input',1,'P')
      | port_label('output',1,'m')
      | port_label('Rconn',1,'A')
      | port_label('Rconn',2,'B')
      | port_label('Rconn',3,'C')
  "Three-Phase Breaker " : powerlib/Elements/Three-Phase Breaker  InitialState=closed  SwitchA=on  SwitchB=on  SwitchC=on  SwitchTimes=[T_Disconnect T_Reconnect]  External=off  BreakerResistance=0.0001  SnubberResistance=1e6  SnubberCapacitance=inf  Measurements=None
      settings: SourceProductName=Simscape Electrical
  Wind Turbine : Subsystem  mask(Grid-Connected Wind Turbine (PQ Model)){Vn=4160, Fn=60, P0=.05*4000e3}
      mask prompts: Vn "Nominal L-L Voltage [Vrms]"; Fn "Nominal Frequency [Hz]"; P0 "Initial Power [W]"
      mask help:
      | This block models a grid-connected wind turbine using the Three-Phase Dynamic Load block. This is a system-level model that does not contain any power electronics, but is useful for load flow, phasor, and hybrid phasor-EMT simulations. The input to this block is the power output of the grid connected wind turbine, not wind speed.
      |
      | For more detailed wind turbine models, consider the available blocks in the Renewables library. Consider using this PQ Model to perform load flow studies and switch to a more detailed model when full EMT studies are required.
      |
      | Note: The wind turbine power must be specified for use for Load Flow analysis.
      mask init:
      | % P0 = Irr0*TotalArea*Efficiency/100;
      | P0 = -P0;
      mask Display:
      | image(imread('eolienne.bmp'))
      | color('white')
      | port_label('input',1,'P')
      | port_label('output',1,'m')
      | port_label('Rconn',1,'A')
      | port_label('Rconn',2,'B')
      | port_label('Rconn',3,'C')
  XFM-1 4.16 kV /480 V : powerlib/Elements/Three-Phase Transformer (Two Windings)  Winding1Connection=Yg  Winding2Connection=Yg  CoreType=Three single-phase transformers  SetSaturation=off  Hysteresis=off  DataFile='hysteresis'  SetInitialFlux=off  Measurements=None  UNITS=pu  NominalPower=[ 500e3 , 60 ]  Winding1=[4160 0.011 0.02]  Winding2=[480 0 0]  Rm=500  Lm=500  L0=0.5  Saturation=[0 0;0.0024 1.2;1 1.52]  InitialFluxes=[0.8 -0.8 0.7]  BreakLoop=off  DiscreteSolver=Trapezoidal iterative  DataType=off  TransfoNumber=1
      settings: SourceProductName=Simscape Electrical
  YT SOLAR PROFILE : Subsystem
  YT WIND PROFILE : Subsystem
  powergui : powerlib/powergui  Priority=1  SimulationMode=Phasor  SampleTime=50e-6  frequency=60  Iterations=50  frequencyindice=60  Pbase=100e3  ErrMax=0.0001  UnitsV=kV  UnitsW=kW  buscounter=0  FunctionMessages=off  echomessages=off  EnableUseOfTLC=off  CurrentSourceSwitches=off  DisableSnubberDevices=off  DisableRonSwitches=off  DisableVfSwitches=off  DisplayEquations=off  AutomaticDiscreteSolvers=off  SolverType=Tustin/Backward Euler (TBE)  Interpol=off  ExternalGateDelay=off  methode=off  Ts=0  x0status=blocks  SPID=off  SwTol=0  HookPort=off  NonlinearTolerance=1e-4  nMaxIteration=100  ContinueOnMaxIteration=off  RestoreLinks=warning  ResistiveCurrentMeasurement=off  Frange=[0:2:500]  Ylog=off  Xlog=on  ShowGrid=off  save=off  variable=ZData  structure=0  ZoomFFT=on  StartTime=0.0  cycles=1  DisplayStyle=1  fundamental=60  FreqAxis=off  MaxFrequency=1000  frequencyindicesteady=1  RmsSteady=1  display=off
      settings: SourceProductName=Simscape Electrical
  Scope : Scope
  Scope1 : Scope
  wires:
  .2/1 -> Diesel Generator1/1(wref (pu)), Diesel Generator1/2(Vref (pu))
  MB WIND PROFILE/2(Power) -> Wind Turbine/1(P)
  MB SOLAR PROFILE/2(Power) -> Solar Array/1(P)
  connections:
  Load Flow Bar5/LConn2 -- 2/RConn2 -- 671 Yg PQ/LConn2 -- 632-671/RConn2
  Load Flow Bar5/LConn1 -- 2/RConn1 -- 671 Yg PQ/LConn1 -- 632-671/RConn1
  Load Flow Bar5/LConn3 -- 2/RConn3 -- 671 Yg PQ/LConn3 -- 632-671/RConn3
  Load Flow Bar7/LConn1 -- 4/RConn1 -- 675 Yg Z/LConn1 -- 675 Yg PQ/LConn1
  Load Flow Bar7/LConn2 -- 4/RConn2 -- 675 Yg Z/LConn2 -- 675 Yg PQ/LConn2
  Load Flow Bar7/LConn3 -- 4/RConn3 -- 675 Yg Z/LConn3 -- 675 Yg PQ/LConn3
  Load Flow Bar10/RConn1 -- 684-611/LConn1
  Load Flow Bar1/LConn1 -- 632-633/RConn1
  Load Flow Bar1/LConn2 -- 632-633/RConn2
  Load Flow Bar1/LConn3 -- 632-633/RConn3
  Load Flow Bar2/LConn1 -- XFM-1 4.16 kV /480 V/RConn1
  Load Flow Bar2/LConn2 -- XFM-1 4.16 kV /480 V/RConn2
  Load Flow Bar2/LConn3 -- XFM-1 4.16 kV /480 V/RConn3
  Load Flow Bar3/RConn1 -- PQ/LConn1 -- 632-645/LConn1
  Load Flow Bar3/RConn2 -- 632-645/LConn2
  Load Flow Bar6/LConn1 -- 692-675/LConn1
  Load Flow Bar6/LConn2 -- 692-675/LConn2
  Load Flow Bar6/LConn3 -- 692-675/LConn3
  671 D PQ/LConn1 -- 671/RConn1 -- Breaker/LConn1 -- 671-684/RConn1 -- 671-680/LConn1
  671 D PQ/LConn2 -- 671/RConn2 -- Breaker/LConn2 -- 671-680/LConn2
  671-680/LConn3 -- 671/RConn3 -- 671 D PQ/LConn3 -- 671-684/RConn2 -- Breaker/LConn3
  692 D I/LConn1 -- 692/LConn1 -- Breaker/RConn1
  692 D I/LConn2 -- 692/LConn2 -- Breaker/RConn2
  692 D I/LConn3 -- 692/LConn3 -- Breaker/RConn3
  Load Flow Bar4/RConn1 -- 645-646/LConn1
  Load Flow Bar4/RConn2 -- 645-646/LConn2
  Load Flow Bar11/LConn1 -- 684-652/RConn1
  Load Flow Bar9/RConn1 -- 671-684/LConn1
  Load Flow Bar9/RConn2 -- 671-684/LConn2
  Ground/LConn1 -- PQ/RConn1
  Ground2/LConn1 -- 611 Z/RConn1
  611 I/LConn1 -- 611 Z/LConn1 -- 611 (1phase measure)/RConn1
  Ground1/LConn1 -- "652  Z "/RConn1
  Ground3/LConn1 -- 611 I/RConn1
  692/RConn1 -- Load Flow Bar6/RConn1
  692/RConn2 -- Load Flow Bar6/RConn2
  692/RConn3 -- Load Flow Bar6/RConn3
  633/LConn1 -- Load Flow Bar1/RConn1
  633/LConn2 -- Load Flow Bar1/RConn2
  633/LConn3 -- Load Flow Bar1/RConn3
  633/RConn3 -- XFM-1 4.16 kV /480 V/LConn3
  633/RConn2 -- XFM-1 4.16 kV /480 V/LConn2
  633/RConn1 -- XFM-1 4.16 kV /480 V/LConn1
  671/LConn1 -- Load Flow Bar5/RConn1
  671/LConn2 -- Load Flow Bar5/RConn2
  671/LConn3 -- Load Flow Bar5/RConn3
  634/LConn1 -- Load Flow Bar2/RConn1
  634/LConn2 -- Load Flow Bar2/RConn2
  634/LConn3 -- Load Flow Bar2/RConn3
  634/RConn3 -- " 634 Yg PQ "/LConn3
  634/RConn2 -- " 634 Yg PQ "/LConn2
  634/RConn1 -- " 634 Yg PQ "/LConn1
  "675 "/LConn1 -- 692-675/RConn1
  "675 "/LConn2 -- 692-675/RConn2
  "675 "/LConn3 -- 692-675/RConn3
  "675 "/RConn1 -- Load Flow Bar7/RConn1
  "675 "/RConn2 -- Load Flow Bar7/RConn2
  "675 "/RConn3 -- Load Flow Bar7/RConn3
  680/LConn1 -- 671-680/RConn1
  680/LConn2 -- 671-680/RConn2
  680/LConn3 -- 671-680/RConn3
  680/RConn1 -- Load Flow Bar8/LConn1
  680/RConn2 -- Load Flow Bar8/LConn2
  680/RConn3 -- Load Flow Bar8/LConn3
  684 (2phase measure)/LConn1 -- Load Flow Bar9/LConn1
  684 (2phase measure)/RConn1 -- 684-611/RConn1
  684 (2phase measure)/LConn2 -- Load Flow Bar9/LConn2
  684 (2phase measure)/RConn2 -- 684-652/LConn1
  645 (2phase measure)1/LConn1 -- Load Flow Bar3/LConn1
  645 (2phase measure)1/LConn2 -- Load Flow Bar3/LConn2
  645 (2phase measure)1/RConn1 -- 645-646/RConn1
  645 (2phase measure)1/RConn2 -- 645-646/RConn2
  646 (2phase measure)2/LConn1 -- Load Flow Bar4/LConn1
  646 (2phase measure)2/LConn2 -- Load Flow Bar4/LConn2
  646 (2phase measure)2/RConn2 -- 646_Z/RConn1
  646 (2phase measure)2/RConn1 -- 646_Z/LConn1
  611 (1phase measure)/LConn1 -- Load Flow Bar10/LConn1
  652 (1phase measure)/LConn1 -- Load Flow Bar11/RConn1
  652 (1phase measure)/RConn1 -- "652  Z "/LConn1
  "Three-Phase Breaker "/RConn1 -- Load Flow Bar/LConn1
  "Three-Phase Breaker "/RConn2 -- Load Flow Bar/LConn2
  "Three-Phase Breaker "/RConn3 -- Load Flow Bar/LConn3
  Load Flow Bar/RConn1 -- 632/LConn1
  Load Flow Bar/RConn2 -- 632/LConn2
  Load Flow Bar/RConn3 -- 632/LConn3
  3/RConn1 -- "Three-Phase Breaker "/LConn1
  3/RConn2 -- "Three-Phase Breaker "/LConn2
  3/RConn3 -- "Three-Phase Breaker "/LConn3
  3/LConn1 -- Load Flow Bar12/RConn1
  3/LConn2 -- Load Flow Bar12/RConn2
  3/LConn3 -- Load Flow Bar12/RConn3
  4160 V swing/RConn1 -- Load Flow Bar12/LConn1
  4160 V swing/RConn2 -- Load Flow Bar12/LConn2
  4160 V swing/RConn3 -- Load Flow Bar12/LConn3
  632-645/RConn2 -- 632/RConn3 -- 1/RConn3 -- 632 Yg PQ/LConn3 -- 632-633/LConn3 -- 632-671/LConn3
  632-645/RConn1 -- 1/RConn2 -- 632/RConn2 -- 632 Yg PQ/LConn2 -- 632-671/LConn2 -- 632-633/LConn2
  632-633/LConn1 -- 1/RConn1 -- 632/RConn1 -- 632 Yg PQ/LConn1 -- 632-671/LConn1
  Wind Turbine/RConn1 -- 2/LConn1
  Wind Turbine/RConn2 -- 2/LConn2
  Wind Turbine/RConn3 -- 2/LConn3
  Solar Array/RConn1 -- 4/LConn1
  Solar Array/RConn2 -- 4/LConn2
  Solar Array/RConn3 -- 4/LConn3
  Diesel Generator1/RConn1 -- 1/LConn1
  Diesel Generator1/RConn2 -- 1/LConn2
  Diesel Generator1/RConn3 -- 1/LConn3

== system CurrentSystem2019a/611 (1phase measure) ==
  611 : powerlib/Measurements/Three-Phase V-I Measurement  VoltageMeasurement=phase-to-ground  SetLabelV=on  LabelV=Vabc_611  Vpu=off  VpuLL=off  CurrentMeasurement=yes  SetLabelI=on  LabelI=Iabc_611  Ipu=off  Pbase=100e6  Vbase=4160  OutputType=Complex  PhasorSimulation=on  PSBequivalent=0
      settings: SourceProductName=Simscape Electrical
  Ground4 : powerlib/Elements/Ground  LConnTagsString=a
      settings: SourceProductName=Simscape Electrical
  C : PMIOPort  Side=Left
  c : PMIOPort  Port=2  Side=Right
  connections:
  C/RConn1 -- 611/LConn3
  c/RConn1 -- 611/RConn3
  Ground4/LConn1 -- 611/LConn2 -- 611/LConn1 -- 611/RConn2 -- 611/RConn1

== system CurrentSystem2019a/645 (2phase measure)1 ==
  645 : powerlib/Measurements/Three-Phase V-I Measurement  VoltageMeasurement=phase-to-ground  SetLabelV=on  LabelV=Vabc_645  Vpu=off  VpuLL=off  CurrentMeasurement=yes  SetLabelI=on  LabelI=Iabc_645  Ipu=off  Pbase=100e6  Vbase=4160  OutputType=Complex  PhasorSimulation=on  PSBequivalent=0
      settings: SourceProductName=Simscape Electrical
  Ground4 : powerlib/Elements/Ground  LConnTagsString=a
      settings: SourceProductName=Simscape Electrical
  B : PMIOPort  Side=Left
  c : PMIOPort  Port=2  Side=Right
  C : PMIOPort  Port=3  Side=Left
  b : PMIOPort  Port=4  Side=Right
  connections:
  Ground4/LConn1 -- 645/RConn1 -- 645/LConn1
  C/RConn1 -- 645/LConn3
  B/RConn1 -- 645/LConn2
  b/RConn1 -- 645/RConn2
  c/RConn1 -- 645/RConn3

== system CurrentSystem2019a/646 (2phase measure)2 ==
  646 : powerlib/Measurements/Three-Phase V-I Measurement  VoltageMeasurement=phase-to-ground  SetLabelV=on  LabelV=Vabc_646  Vpu=off  VpuLL=off  CurrentMeasurement=yes  SetLabelI=on  LabelI=Iabc_646  Ipu=off  Pbase=100e6  Vbase=4160  OutputType=Complex  PhasorSimulation=on  PSBequivalent=0
      settings: SourceProductName=Simscape Electrical
  Ground4 : powerlib/Elements/Ground  LConnTagsString=a
      settings: SourceProductName=Simscape Electrical
  B : PMIOPort  Side=Left
  c : PMIOPort  Port=2  Side=Right
  C : PMIOPort  Port=3  Side=Left
  b : PMIOPort  Port=4  Side=Right
  connections:
  Ground4/LConn1 -- 646/LConn1 -- 646/RConn1
  C/RConn1 -- 646/LConn3
  B/RConn1 -- 646/LConn2
  b/RConn1 -- 646/RConn2
  c/RConn1 -- 646/RConn3

== system CurrentSystem2019a/652 (1phase measure) ==
  "652 " : powerlib/Measurements/Three-Phase V-I Measurement  VoltageMeasurement=phase-to-ground  SetLabelV=on  LabelV=Vabc_652  Vpu=off  VpuLL=off  CurrentMeasurement=yes  SetLabelI=on  LabelI=Iabc_652  Ipu=off  Pbase=100e6  Vbase=4160  OutputType=Complex  PhasorSimulation=on  PSBequivalent=0
      settings: SourceProductName=Simscape Electrical
  Ground4 : powerlib/Elements/Ground  LConnTagsString=a
      settings: SourceProductName=Simscape Electrical
  A : PMIOPort  Side=Left
  a : PMIOPort  Port=2  Side=Right
  connections:
  a/RConn1 -- "652 "/RConn1
  A/RConn1 -- "652 "/LConn1
  "652 "/RConn3 -- "652 "/RConn2 -- "652 "/LConn3 -- "652 "/LConn2 -- Ground4/LConn1

== system CurrentSystem2019a/684 (2phase measure) ==
  684 : powerlib/Measurements/Three-Phase V-I Measurement  VoltageMeasurement=phase-to-ground  SetLabelV=on  LabelV=Vabc_684  Vpu=off  VpuLL=off  CurrentMeasurement=yes  SetLabelI=on  LabelI=Iabc_684  Ipu=off  Pbase=100e6  Vbase=4160  OutputType=Complex  PhasorSimulation=on  PSBequivalent=0
      settings: SourceProductName=Simscape Electrical
  Ground4 : powerlib/Elements/Ground  LConnTagsString=a
      settings: SourceProductName=Simscape Electrical
  A : PMIOPort  Side=Left
  c : PMIOPort  Port=2  Side=Right
  C : PMIOPort  Port=3  Side=Left
  a : PMIOPort  Port=4  Side=Right
  connections:
  Ground4/LConn1 -- 684/RConn2 -- 684/LConn2
  684/LConn1 -- A/RConn1
  684/LConn3 -- C/RConn1
  684/RConn3 -- c/RConn1
  684/RConn1 -- a/RConn1

== system CurrentSystem2019a/AB SOLAR PROFILE ==
  Add : Sum  Inputs=++++++++++++
  Apr : Step  Time=3*Yearsec  After=129-121  SampleTime=0
  Aug : Step  Time=7*Yearsec  After=123-128  SampleTime=0
  Dec : Step  Time=11*Yearsec  After=62-75  SampleTime=0
  Egen : Gain  Gain=ABSOLARCap
  Feb : Step  Time=1*Yearsec  After=101  SampleTime=0
  Jan : Step  Time=1*Yearsec  Before=74  After=0  SampleTime=0
  Jul : Step  Time=6*Yearsec  After=128-124  SampleTime=0
  Jun : Step  Time=5*Yearsec  After=124-120  SampleTime=0
  Mar : Step  Time=2*Yearsec  After=121-101  SampleTime=0
  May : Step  Time=4*Yearsec  After=120-129  SampleTime=0
  Nov : Step  Time=10*Yearsec  After=75-104  SampleTime=0
  Oct : Step  Time=9*Yearsec  After=104-115  SampleTime=0
  Pgen : Gain  Gain=(1/(30*24))*ABSOLARCap
  Sept : Step  Time=8*Yearsec  After=115-123  SampleTime=0
  Energy : Outport
  Power : Outport  Port=2
  wires:
  Dec/1 -> Add/12
  Sept/1 -> Add/9
  Jun/1 -> Add/6
  Nov/1 -> Add/11
  Aug/1 -> Add/8
  Mar/1 -> Add/3
  May/1 -> Add/5
  Apr/1 -> Add/4
  Jan/1 -> Add/1
  Oct/1 -> Add/10
  Jul/1 -> Add/7
  Feb/1 -> Add/2
  Pgen/1 -> Power/1
  Egen/1 -> Energy/1
  Add/1 -> Egen/1, Pgen/1

== system CurrentSystem2019a/AB WIND PROFILE ==
  Add : Sum  Inputs=++++++++++++
  Apr : Step  Time=3*Yearsec  After=24-0  SampleTime=0
  Aug : Step  Time=7*Yearsec  After=1.2-2.88  SampleTime=0
  Dec : Step  Time=11*Yearsec  After=0-0  SampleTime=0
  Egen : Gain  Gain=ABWindCap
  Feb : Step  Time=1*Yearsec  After=0  SampleTime=0
  Jan : Step  Time=1*Yearsec  After=0  SampleTime=0
  Jul : Step  Time=6*Yearsec  After=2.88-45.6  SampleTime=0
  Jun : Step  Time=5*Yearsec  After=45.6-24  SampleTime=0
  Mar : Step  Time=2*Yearsec  After=0-0  SampleTime=0
  May : Step  Time=4*Yearsec  After=24-24  SampleTime=0
  Nov : Step  Time=10*Yearsec  After=0-10.8  SampleTime=0
  Oct : Step  Time=9*Yearsec  After=10.8-0.48  SampleTime=0
  Pgen : Gain  Gain=(1/(30*24))*ABWindCap
  Sept : Step  Time=8*Yearsec  After=0.48-1.2  SampleTime=0
  Energy : Outport
  Power : Outport  Port=2
  wires:
  Dec/1 -> Add/12
  Sept/1 -> Add/9
  Jun/1 -> Add/6
  Nov/1 -> Add/11
  Aug/1 -> Add/8
  Mar/1 -> Add/3
  May/1 -> Add/5
  Apr/1 -> Add/4
  Jan/1 -> Add/1
  Oct/1 -> Add/10
  Jul/1 -> Add/7
  Feb/1 -> Add/2
  Pgen/1 -> Power/1
  Egen/1 -> Energy/1
  Add/1 -> Egen/1, Pgen/1

== system CurrentSystem2019a/BC SOLAR PROFILE ==
  Add : Sum  Inputs=++++++++++++
  Apr : Step  Time=3*Yearsec  After=99-84  SampleTime=0
  Aug : Step  Time=7*Yearsec  After=118-120  SampleTime=0
  Dec : Step  Time=11*Yearsec  After=37-44  SampleTime=0
  Egen : Gain  Gain=BCSOLARCap
  Feb : Step  Time=1*Yearsec  After=58  SampleTime=0
  Jan : Step  Time=1*Yearsec  Before=40  After=0  SampleTime=0
  Jul : Step  Time=6*Yearsec  After=120-110  SampleTime=0
  Jun : Step  Time=5*Yearsec  After=110-104  SampleTime=0
  Mar : Step  Time=2*Yearsec  After=84-58  SampleTime=0
  May : Step  Time=4*Yearsec  After=104-99  SampleTime=0
  Nov : Step  Time=10*Yearsec  After=44-74  SampleTime=0
  Oct : Step  Time=9*Yearsec  After=74-113  SampleTime=0
  Pgen : Gain  Gain=(1/(30*24))*BCSOLARCap
  Sept : Step  Time=8*Yearsec  After=113-118  SampleTime=0
  Energy : Outport
  Power : Outport  Port=2
  wires:
  Dec/1 -> Add/12
  Sept/1 -> Add/9
  Jun/1 -> Add/6
  Nov/1 -> Add/11
  Aug/1 -> Add/8
  Mar/1 -> Add/3
  May/1 -> Add/5
  Apr/1 -> Add/4
  Jan/1 -> Add/1
  Oct/1 -> Add/10
  Jul/1 -> Add/7
  Feb/1 -> Add/2
  Pgen/1 -> Power/1
  Egen/1 -> Energy/1
  Add/1 -> Egen/1, Pgen/1

== system CurrentSystem2019a/BC WIND PROFILE ==
  Add : Sum  Inputs=++++++++++++
  Apr : Step  Time=3*Yearsec  After=12-9.6  SampleTime=0
  Aug : Step  Time=7*Yearsec  After=0-0  SampleTime=0
  Dec : Step  Time=11*Yearsec  After=2.4-0.48  SampleTime=0
  Egen : Gain  Gain=BCWindCap
  Feb : Step  Time=1*Yearsec  After=14.4  SampleTime=0
  Jan : Step  Time=1*Yearsec  Before=4.8  After=0  SampleTime=0
  Jul : Step  Time=6*Yearsec  After=0-9.6  SampleTime=0
  Jun : Step  Time=5*Yearsec  After=9.6-0  SampleTime=0
  Mar : Step  Time=2*Yearsec  After=9.6-14.4  SampleTime=0
  May : Step  Time=4*Yearsec  After=0-12  SampleTime=0
  Nov : Step  Time=10*Yearsec  After=0.48-0  SampleTime=0
  Oct : Step  Time=9*Yearsec  After=0-0  SampleTime=0
  Pgen : Gain  Gain=(1/(30*24))*BCWindCap
  Sept : Step  Time=8*Yearsec  After=0-0  SampleTime=0
  Energy : Outport
  Power : Outport  Port=2
  wires:
  Dec/1 -> Add/12
  Sept/1 -> Add/9
  Jun/1 -> Add/6
  Nov/1 -> Add/11
  Aug/1 -> Add/8
  Mar/1 -> Add/3
  May/1 -> Add/5
  Apr/1 -> Add/4
  Jan/1 -> Add/1
  Oct/1 -> Add/10
  Jul/1 -> Add/7
  Feb/1 -> Add/2
  Pgen/1 -> Power/1
  Egen/1 -> Energy/1
  Add/1 -> Egen/1, Pgen/1
